simulink model "P2_Q2"  (R2023a)
settings: Solver=VariableStepAuto  StartTime=0.0  StopTime=50  RelTol=1e-3
libraries: simulink x2
settings Model: Creator=asus  LastModifiedBy=asus

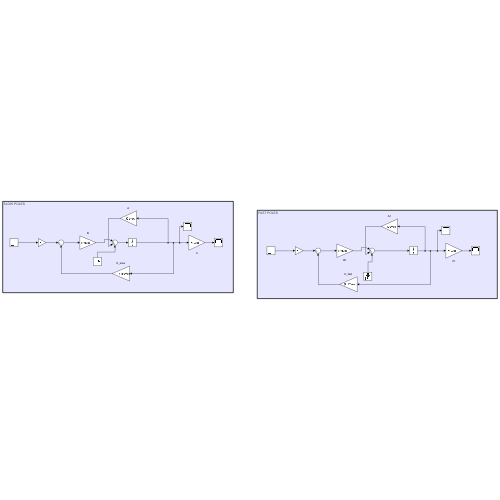
[thumbnail: Simulink's stored preview of the top-level diagram]
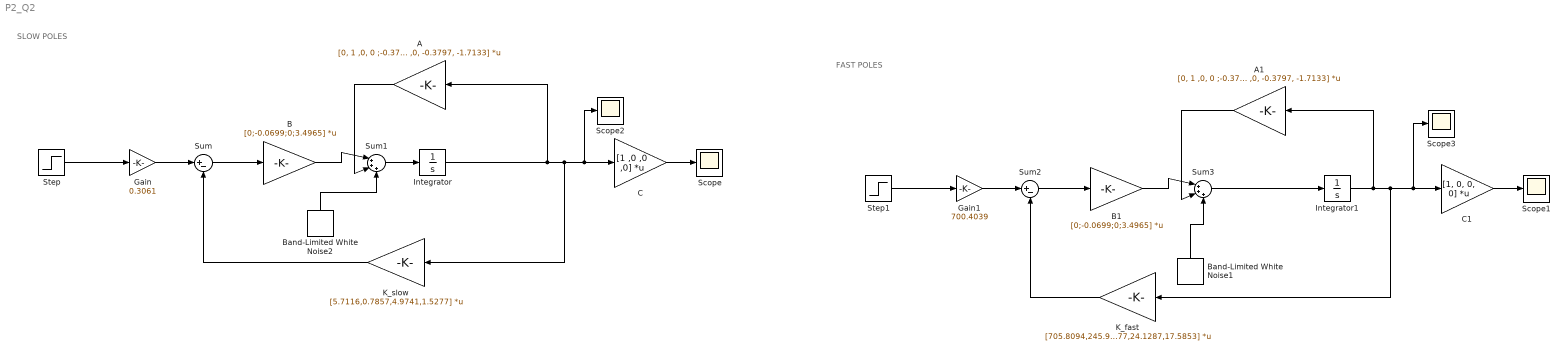
== system P2_Q2 ==
  note: FAST POLES
  note: SLOW POLES
  A : Gain  Gain=[0, 1 ,0, 0 ;-0.378 ,0 ,7.0147 ,0.0343;0, 0, 0, 1; 18.9001 ,0, -0.3797, -1.7133]  Multiplication=Matrix(K*u) (u vector)
  A1 : Gain  Gain=[0, 1 ,0, 0 ;-0.378 ,0 ,7.0147 ,0.0343;0, 0, 0, 1; 18.9001 ,0, -0.3797, -1.7133]  Multiplication=Matrix(K*u) (u vector)
  B : Gain  Gain=[0;-0.0699;0;3.4965]  Multiplication=Matrix(K*u) (u vector)
  B1 : Gain  Gain=[0;-0.0699;0;3.4965]  Multiplication=Matrix(K*u) (u vector)
  Band-Limited White Noise1 : simulink/Sources/Band-Limited White Noise  Cov=[1e-5; 1e-5; 1e-5; 1e-5]  Ts=10  seed=[456; 5000; 2000; 1000]
  Band-Limited White Noise2 : simulink/Sources/Band-Limited White Noise  Cov=[1e-5; 1e-5; 1e-5; 1e-5]  Ts=10  seed=[456; 5000; 2000; 1000]
  C : Gain  Gain=[1 ,0 ,0 ,0]  Multiplication=Matrix(K*u) (u vector)
  C1 : Gain  Gain=[1, 0, 0, 0]  Multiplication=Matrix(K*u) (u vector)
  Gain : Gain  Gain=0.3061
  Gain1 : Gain  Gain=700.4039
  Integrator : Integrator
  Integrator1 : Integrator
  K_fast : Gain  Gain=[705.8094,245.9577,24.1287,17.5853]  Multiplication=Matrix(K*u) (u vector)
  K_slow : Gain  Gain=[5.7116,0.7857,4.9741,1.5277]  Multiplication=Matrix(K*u) (u vector)
  Scope{,1..3} (4 alike) : Scope
  Step : Step  Time=0  After=0.1  SampleTime=0
  Step1 : Step  Time=0  After=0.1  SampleTime=0
  Sum : Sum  Inputs=|+-
  Sum1 : Sum  Inputs=|+++
  Sum2 : Sum  Inputs=|+-
  Sum3 : Sum  Inputs=|+++
  wires:
  C1/1 -> Scope1/1
  Sum3/1 -> Integrator1/1
  K_slow/1 -> Sum/2
  Gain/1 -> Sum/1
  Sum1/1 -> Integrator/1
  Integrator1/1 -> A1/1, Scope3/1, C1/1, K_fast/1
  Gain1/1 -> Sum2/1
  Step/1 -> Gain/1
  Sum2/1 -> B1/1
  B/1 -> Sum1/1
  Sum/1 -> B/1
  B1/1 -> Sum3/1
  A/1 -> Sum1/2
  Integrator/1 -> Scope2/1, C/1, K_slow/1, A/1
  C/1 -> Scope/1
  K_fast/1 -> Sum2/2
  A1/1 -> Sum3/2
  Step1/1 -> Gain1/1
  Band-Limited White Noise2/1 -> Sum1/3
  Band-Limited White Noise1/1 -> Sum3/3
